simulink model "Modelo_motor_dc"  (R2020b)
settings: Solver=VariableStepAuto  StartTime=0.0  StopTime=20  RelTol=1e-3
settings Model: Creator=Marce  LastModifiedBy=Marce

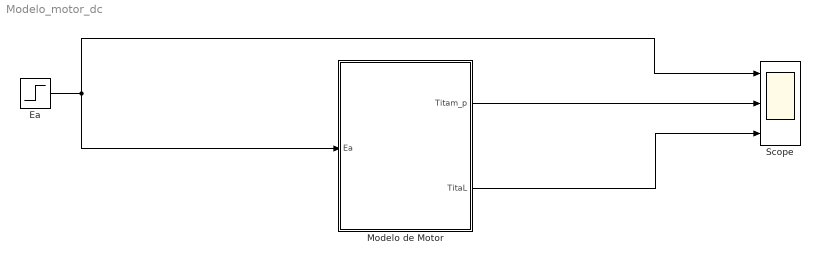
== system Modelo_motor_dc ==
  Ea : Step  SampleTime=0
  Modelo de Motor : Subsystem  mask{Ra=1, La=1e-3, Kb=2, Kt=5, Jm=12, Dm=10, N1=100, N2=1000}
      mask prompts: Ra "Resistencia de armadura [ohm]"; La "Inductancia de armadura [Hy]"; Kb "Constante de fem [Vseg/rad]"; Kt "Contante de cupla [[Nm/A]"; Jm "Momento de inercia total [Kgm2]"; Dm "Friccion total [Nmseg/rad]"; N1 "Numero de dientes engranaje conductor"; N2 "Numero de dientes engranaje conducido"
      mask DialogControl DescTextVar Prompt: Parametros motor
  Scope : Scope  NumInputPorts=3
  wires:
  Ea/1 -> Modelo de Motor/1(Ea), Scope/1
  Modelo de Motor/1(Titam_p) -> Scope/2
  Modelo de Motor/2(TitaL) -> Scope/3

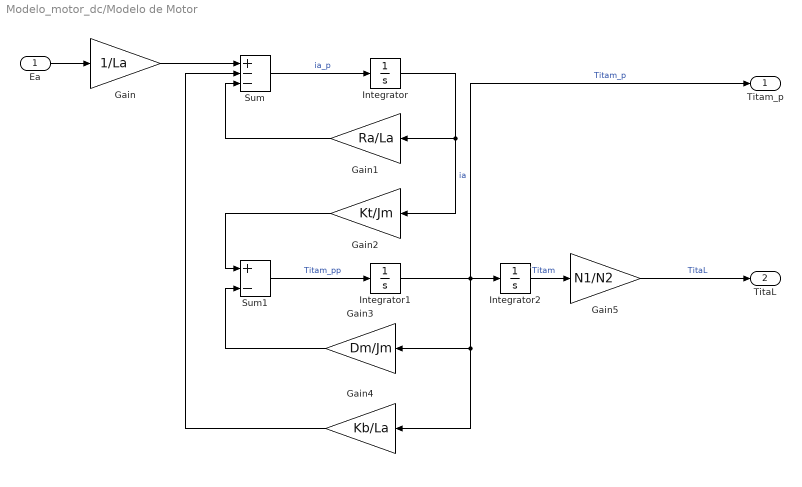
== system Modelo_motor_dc/Modelo de Motor ==
  Ea : Inport
  Gain : Gain  Gain=1/La
  Gain1 : Gain  Gain=Ra/La
  Gain2 : Gain  Gain=Kt/Jm
  Gain3 : Gain  Gain=Dm/Jm
  Gain4 : Gain  Gain=Kb/La
  Gain5 : Gain  Gain=N1/N2
  Integrator : Integrator
  Integrator1 : Integrator
  Integrator2 : Integrator
  Sum : Sum  Inputs=+--
  Sum1 : Sum  Inputs=+-
  Titam_p : Outport
  TitaL : Outport  Port=2
  wires:
  Gain1/1 -> Sum/3
  Sum/1 -> Integrator/1  "ia_p"
  Integrator2/1 -> Gain5/1  "Titam"
  Gain2/1 -> Sum1/1
  Integrator1/1 -> Titam_p/1, Gain3/1, Gain4/1, Integrator2/1  "Titam_p"
  Integrator/1 -> Gain1/1, Gain2/1  "ia"
  Gain4/1 -> Sum/2
  Gain/1 -> Sum/1
  Sum1/1 -> Integrator1/1  "Titam_pp"
  Gain3/1 -> Sum1/2
  Ea/1 -> Gain/1
  Gain5/1 -> TitaL/1  "TitaL"
